simulink model "logibone_motorcontrol1"  (R2014b)
settings: Solver=FixedStepDiscrete  StartTime=0.0  StopTime=inf  RelTol=1e-3
libraries: simulink x2
settings Model: ModifiedByFormat=The MathWorks Inc.  SimulationMode=external  ExtModeTrigDuration=200  ExtModeLogAll=off  Creator=The MathWorks Inc.  LastModifiedBy=The MathWorks Inc.
settings OptimizationCC: OptimizeModelRefInitCode=on  LifeSpan=Inf  MaxStackSize=64
settings DebuggingCC: UnderspecifiedInitializationDetection=Classic  MergeDetectMultiDrivingBlocksExec=none
settings HardwareCC: ProdLargestAtomicInteger=Long  ProdLargestAtomicFloat=Double  ProdEndianess=LittleEndian  ProdHWDeviceType=ARM Compatible->ARM Cortex
settings RTWCC: SystemTargetFile=ert.tlc  TemplateMakefile=ert_default_tmf  Description=Embedded Coder  ProcessScript=ert_make_rtw_hook  Toolchain=Linaro Toolchain v4.8
settings CodeAppCC: IgnoreCustomStorageClasses=off
settings ERTTargetCC: ExtMode=on  ExtModeMexArgs='arm.dhcp.mathworks.com' 1 17725 5

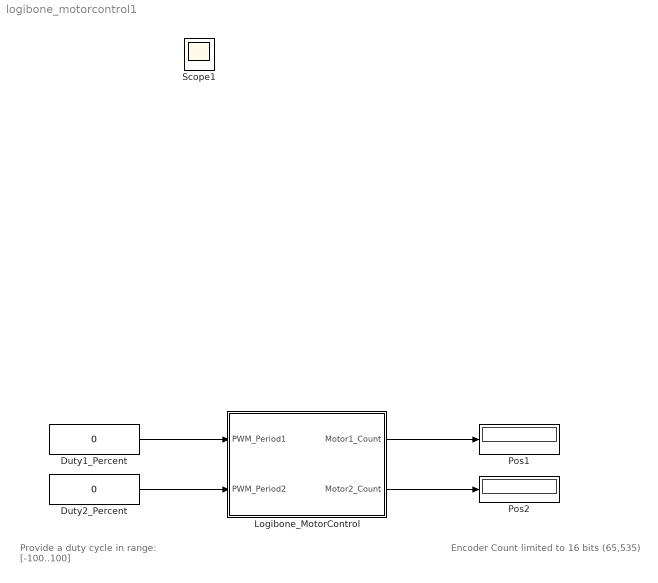
== system logibone_motorcontrol1 ==
  note: Encoder Count limited to 16 bits (65,535)
  note: Provide a duty cycle in range:
      | [-100..100]
  Duty1_Percent : Constant  Value=0  OutDataTypeStr=single  SampleTime=0.1
  Duty2_Percent : Constant  Value=0  OutDataTypeStr=single
  Logibone_MotorControl : Subsystem
  Pos1 : Display
  Pos2 : Display
  Scope1 : Scope  NumInputPorts=2
      settings: YMin=8900~3400  YMax=9800~4400  ScrollMode=on
  wires:
  Duty1_Percent/1 -> Logibone_MotorControl/1(PWM_Period1)
  Duty2_Percent/1 -> Logibone_MotorControl/2(PWM_Period2)
  Logibone_MotorControl/1(Motor1_Count) -> Pos1/1
  Logibone_MotorControl/2(Motor2_Count) -> Pos2/1

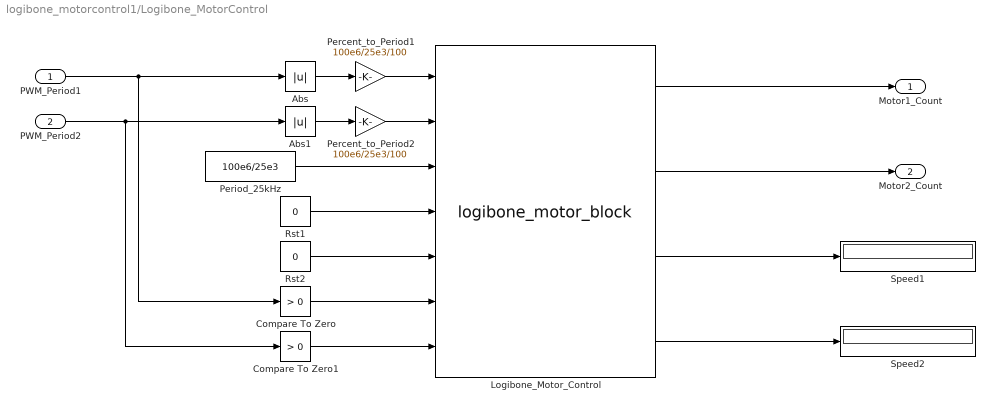
== system logibone_motorcontrol1/Logibone_MotorControl ==
  PWM_Period1 : Inport
  PWM_Period2 : Inport  Port=2
  Abs : Abs
  Abs1 : Abs
  Compare To Zero : simulink/Logic and Bit Operations/Compare To Zero  relop=>  OutDataTypeStr=boolean
  Compare To Zero1 : simulink/Logic and Bit Operations/Compare To Zero  relop=>  OutDataTypeStr=boolean
  Logibone_Motor_Control : S-Function  InitFcn=try, set_param(gcb,'FunctionName','logibone_motor_block'), end  FunctionName=logibone_motor_block  SFunctionModules=logibone_motor_block_wrapper  EnableBusSupport=off  mask(S-Function Builder){}
      mask help: Simulink:masks:SFunctionBuilder_MD
      mask init:
      | val = [[.9  0.75 0.75 1 1 .9 .9 1]',[1 1 0.75 0.75 .9 .9 1 .9]'];try , sys = get_param(gcb,'SfunBuilderFcnName');if isempty(sys), sys = get_param(gcb,'FunctionName'); end,catch, sys = get_param(gcb,'FunctionName'); end
      settings: CopyFcn=set_param(gcbh,'LinkStatus','none')  PreSaveFcn=try, set_param(gcb,'FunctionName','logibone_motor_block'), end  OpenFcn=sfunctionwizard(gcbh)
      mask Display: plot(val(:,1),val(:,2)),disp(sys), port_label('input',1,'duty1'), port_label('input',2,'duty2'), port_label('input',3,'period'), port_label('input',4,'reset_cnt1'), port_label('input',5,'reset_cnt2'), port_label('input',6,'dir1'), port_label('input',7,'dir2'), port_label('output',1,'cnt1'), port_label('output',2,'cnt2'), port_label('output',3,'spd1'), port_label('output',4,'spd2')
  Percent_to_Period1 : Gain  Gain=100e6/25e3/100  OutDataTypeStr=uint16
  Percent_to_Period2 : Gain  Gain=100e6/25e3/100  OutDataTypeStr=uint16
  Period_25kHz : Constant  Value=100e6/25e3  OutDataTypeStr=Inherit: Inherit via back propagation
  Rst1 : Constant  Value=0  OutDataTypeStr=boolean
  Rst2 : Constant  Value=0  OutDataTypeStr=boolean
  Speed1 : Display
      settings: Format=hex (Stored Integer)
  Speed2 : Display
      settings: Format=hex (Stored Integer)
  Motor1_Count : Outport
  Motor2_Count : Outport  Port=2
  wires:
  Percent_to_Period1/1 -> Logibone_Motor_Control/1
  Percent_to_Period2/1 -> Logibone_Motor_Control/2
  Rst2/1 -> Logibone_Motor_Control/5
  Rst1/1 -> Logibone_Motor_Control/4
  PWM_Period1/1 -> Compare To Zero/1, Abs/1
  Compare To Zero1/1 -> Logibone_Motor_Control/7
  Period_25kHz/1 -> Logibone_Motor_Control/3
  Logibone_Motor_Control/3 -> Speed1/1
  Logibone_Motor_Control/1 -> Motor1_Count/1
  Logibone_Motor_Control/2 -> Motor2_Count/1
  Logibone_Motor_Control/4 -> Speed2/1
  Compare To Zero/1 -> Logibone_Motor_Control/6
  PWM_Period2/1 -> Compare To Zero1/1, Abs1/1
  Abs/1 -> Percent_to_Period1/1
  Abs1/1 -> Percent_to_Period2/1
